simulink model "clickpseudoinv"  (R2024a)
settings: Solver=VariableStepAuto  StartTime=0.0  StopTime=100  RelTol=1e-3
model workspace (MAT data in the model file):
  q0 = [25 32 20 14]
  qo = [2; 3; 4; 5]
undefined symbols (not defined in the file or in its folder): DiscIntNeverNeededParam
settings Model: Creator=paola  LastModifiedBy=UTENTE
settings RTWCC: GPUComputeCapability=3.5

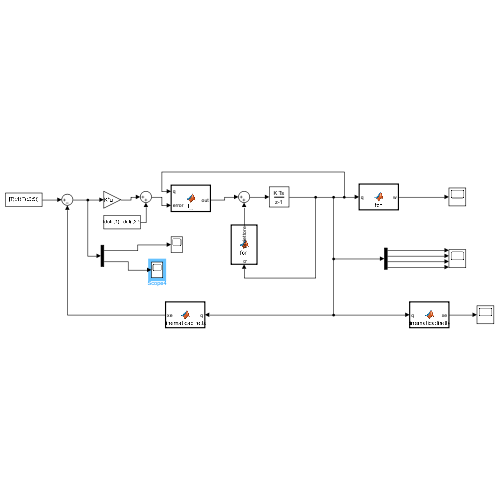
[thumbnail: Simulink's stored preview of the top-level diagram]
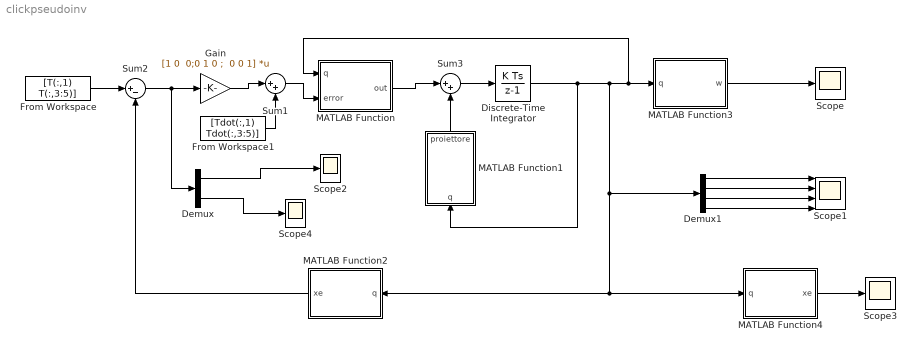
== system clickpseudoinv ==
  Demux : Demux  Outputs=2
  Demux1 : Demux
  Discrete-Time Integrator : DiscreteIntegrator  InitialCondition=[pi/4 pi/6 pi/5 0.5]'  SampleTime=0.001  ICPrevOutput=DiscIntNeverNeededParam  ICPrevScaledInput=DiscIntNeverNeededParam
  From Workspace : FromWorkspace  VariableName=[T(:,1) T(:,3:5)]
  From Workspace1 : FromWorkspace  VariableName=[Tdot(:,1) Tdot(:,3:5)]
  Gain : Gain  Gain="[1 0  0;0 1 0 ;  0 0 1]"  Multiplication=Matrix(K*u)
  MATLAB Function : MATLAB Function  TreatAsAtomicUnit=on
  MATLAB Function1 : MATLAB Function  TreatAsAtomicUnit=on
  MATLAB Function2 : MATLAB Function  TreatAsAtomicUnit=on
  MATLAB Function3 : MATLAB Function  TreatAsAtomicUnit=on
  MATLAB Function4 : MATLAB Function  TreatAsAtomicUnit=on
  Scope{,2..4} (4 alike) : Scope
  Scope1 : Scope  NumInputPorts=4
  Sum1 : Sum  Inputs=|++
  Sum2 : Sum  Inputs=|+-
  Sum3 : Sum  Inputs=|++
  wires:
  Demux1/3 -> Scope1/3
  Demux1/4 -> Scope1/4
  MATLAB Function4/1(xe) -> Scope3/1
  MATLAB Function3/1(w) -> Scope/1
  MATLAB Function2/1(xe) -> Sum2/2
  Demux1/2 -> Scope1/2
  Demux1/1 -> Scope1/1
  Sum3/1 -> Discrete-Time Integrator/1
  Sum2/1 -> Demux/1, Gain/1
  Gain/1 -> Sum1/1
  MATLAB Function1/1(proiettore) -> Sum3/2
  MATLAB Function/1(out) -> Sum3/1
  Demux/1 -> Scope2/1
  Demux/2 -> Scope4/1
  Sum1/1 -> MATLAB Function/2(error)
  Discrete-Time Integrator/1 -> MATLAB Function1/1(q), MATLAB Function/1(q), MATLAB Function3/1(q), Demux1/1, MATLAB Function4/1(q), MATLAB Function2/1(q)
  From Workspace/1 -> Sum2/1
  From Workspace1/1 -> Sum1/2

== matlab function clickpseudoinv/MATLAB Function ==
  data: q input; out output; error input
function out= i_j(q,error)
J=[0.5*cos(q(1))+0.5*cos(q(1)+q(2)) 0.5*cos(q(1)+q(2)) 0 0;
    0 0 -1 0;
    1 1 0 -1];
pinv_Jacobian=J'*inv(J*J');
out = pinv_Jacobian * error;
end

== matlab function clickpseudoinv/MATLAB Function2 ==
  data: q input; xe output
function xe = cinematicadiretta(q)
x_e=[0.5*sin(q(1))+0.5*sin(q(1)+q(2));
        1-q(3);
        q(1)+q(2)-q(4)];
xe=x_e;

== matlab function clickpseudoinv/MATLAB Function3 ==
  data: q input; w output
function w = fcn(q)
w=sqrt( 2*(0.5*cos(q(1)))^2 + 2*0.5*0.5*cos(q(1))*cos(q(1) + q(2)) +2*(0.5*cos(q(1)+q(2)))^2 );
end

== matlab function clickpseudoinv/MATLAB Function4 ==
  data: q input; xe output
function xe = cinematicadiretta(q)
x_e=[0.5*sin(q(1))+0.5*sin(q(1)+q(2));
        1-q(3);
        q(1)+q(2)-q(4)];
xe=x_e;

== matlab function clickpseudoinv/MATLAB Function1 ==
  data: q input; proiettore output
function proiettore = fcn(q)
k0=1500;
a1 = 0.5;
a2 = 0.5;
%k0=0;
I=eye(4);
J=[0.5*cos(q(1))+0.5*cos(q(1)+q(2)) 0.5*cos(q(1)+q(2)) 0 0;
    0 0 -1 0;
    1 1 0 -1];
J_pinv=J'*inv(J*J');
P=I-(J_pinv*J);
% w=sin(q(2))^2;
w=sqrt( 2*(a1*cos(q(1)))^2 + 2*a1*a2*cos(q(1))*cos(q(1) + q(2)) +2*(a2*cos(q(1)+q(2)))^2 );
dwq1=-(2^(1/2)*(2*a2^2*cos(q(1) + q(2))*sin(q(1) + q(2)) + 2*a1^2*cos(q(1))*sin(q(1)) + a1*a2*cos(q(1) + q(2))*sin(q(1)) + a1*a2*sin(q(1) + q(2))*cos(q(1))))/(2*(a1^2*cos(q(1))^2 + a1*a2*cos(q(1) + q(2))*cos(q(1)) + a2^2*cos(q(1) + q(2))^2)^(1/2));
dwq2=-(2^(1/2)*(2*cos(q(1) + q(2))*sin(q(1) + q(2))*a2^2 + a1*sin(q(1) + q(2))*cos(q(1))*a2))/(2*(a1^2*cos(q(1))^2 + a1*a2*cos(q(1) + q(2))*cos(q(1)) + a2^2*cos(q(1) + q(2))^2)^(1/2));
dw=[dwq1; dwq2; 0; 0];
q0_dot=k0*dw;
% q0_dot=k0*[0 2*sin(q(2))*cos(q(2)) 0 0]'
proiettore= P*q0_dot;
end
